simulink model "SimplifiedShiftController5"  (Simulink 8.2)
settings: Solver=ode45  StartTime=0.0  StopTime=10.0  RelTol=1e-3
settings Model: Creator=root  LastModifiedBy=tiwari
settings DataIOCC: SignalLoggingSaveFormat=Dataset
settings OptimizationCC: ExpressionDepthLimit=128
settings DebuggingCC: FcnCallInpInsideContextMsg=EnableAllAsError
settings GRTTargetCC: CombineOutputUpdateFcns=on  GRTInterface=off

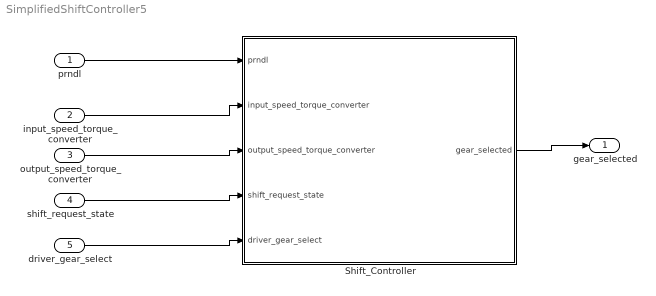
== system SimplifiedShiftController5 ==
  prndl : Inport
  input_speed_torque_converter : Inport  Port=2
  output_speed_torque_converter : Inport  Port=3
  shift_request_state : Inport  Port=4
  driver_gear_select : Inport  Port=5
  Shift_Controller : Subsystem
  gear_selected : Outport
  wires:
  prndl/1 -> Shift_Controller/1(prndl)
  shift_request_state/1 -> Shift_Controller/4(shift_request_state)
  driver_gear_select/1 -> Shift_Controller/5(driver_gear_select)
  output_speed_torque_converter/1 -> Shift_Controller/3(output_speed_torque_converter)
  input_speed_torque_converter/1 -> Shift_Controller/2(input_speed_torque_converter)
  Shift_Controller/1(gear_selected) -> gear_selected/1

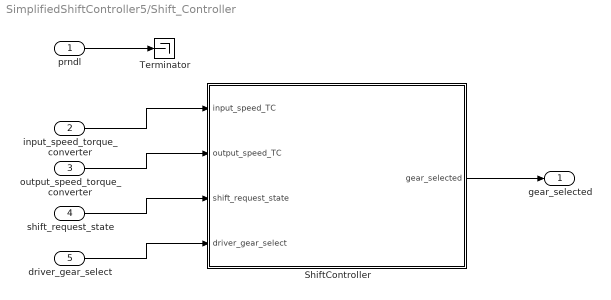
== system SimplifiedShiftController5/Shift_Controller ==
  prndl : Inport
  input_speed_torque_converter : Inport  Port=2
  output_speed_torque_converter : Inport  Port=3
  shift_request_state : Inport  Port=4
  driver_gear_select : Inport  Port=5
  ShiftController : Stateflow chart  TreatAsAtomicUnit=on
  Terminator : Terminator
  gear_selected : Outport
  wires:
  ShiftController/1(gear_selected) -> gear_selected/1
  prndl/1 -> Terminator/1
  input_speed_torque_converter/1 -> ShiftController/1(input_speed_TC)
  output_speed_torque_converter/1 -> ShiftController/2(output_speed_TC)
  shift_request_state/1 -> ShiftController/3(shift_request_state)
  driver_gear_select/1 -> ShiftController/4(driver_gear_select)

== stateflow chart Shift_Controller/ShiftController ==
  settings: description=|
      | <?xml version="1.0" encoding="utf-8"?>
      | <ltlProperties>
      |    <ltlProperty expr="&lt;&gt;((driver_gear_select==6 || driver_gear_select==7)) -&gt; (!((gear_selected /= 0)) U((driver_gear_select==6 || driver_gear_select==7)))" name="AbsenceProperty" type="Absence"/>
      |    <ltlProperty expr="[]((driver_gear_select==6) -&gt; &lt;&gt;(gear_selected &gt;= 1))" name="ResponseProperty" type="Response"/>
      |    <ltlProperty expr="[](((shift_request_state==3 &amp;&amp; driver_gear_select==7)) -&gt; &lt;&gt;(gear_selected == 4))" name="ResponseProperty2" type="Response"/>
      |    <ltlProperty expr="[]((G(shift_request_state==3 &amp;&amp; driver_gear_select==7)) -&gt; &lt;&gt;((gear_selected == 4)))" name="ResponseProperty3" type="Response"/>
      |    <ltlProperty expr="[]((G(driver_gear_select == 1)) -&gt; &lt;&gt;((gear_selected &lt;= 1)))" name="ResponseProperty4" type="Response"/>
      |    <ltlProperty expr="[]((G(driver_gear_select==1)) -&gt; &lt;&gt;((gear_selected &lt;= 2)))" name="ResponseProperty5" type="Response"/>
      | </ltlProperties>
  state gear1
    en:gear_selected=1;
  state lockoutU2
    en: current_time = 0;
    du: current_time += SamplePeriod;
  state gear2
    en: gear_selected = 2;
  state lockoutD1
    en: current_time = 0;
    du: current_time += SamplePeriod;
  state lockoutD2
    en: current_time = 0;
    du: current_time += SamplePeriod;
  state lockoutD3
    en: current_time = 0;
    du: current_time += SamplePeriod;
  state lockoutU3
    en: current_time = 0;
    du: current_time += SamplePeriod;
  state lockoutU4
    en: current_time = 0;
    du:current_time += SamplePeriod;
  state gear3
    en: gear_selected = 3;
  state gear4
    en: gear_selected = 4;
  state gear0
    en:gear_selected=0;
  (default) -> gear0
  gear0 -> gear1 : [(driver_gear_select==6)||(driver_gear_select==7)]
  lockoutD1 -> gear1 : [current_time >= lockout_time]
  gear1 -> lockoutU2 : [(shift_request_state == 3) && (driver_gear_select != 6) && (driver_gear_select != 1)]
  lockoutU2 -> gear2 : [current_time >= lockout_time]
  gear3 -> lockoutD1 [order 3] : [(driver_gear_select == 6) || (driver_gear_select == 1)]
  gear4 -> lockoutD1 [order 2] : [(driver_gear_select == 6) || (driver_gear_select == 1)]
  gear2 -> lockoutD1 [order 2] : [((shift_request_state == 1) && (driver_gear_select != 6) && (driver_gear_select != 1) && (input_speed_TC > output_speed_TC)) || (driver_gear_select==6) || (driver_gear_select==1)]
  lockoutD2 -> gear2 : [current_time >= lockout_time]
  gear2 -> lockoutU3 [order 1] : [(shift_request_state == 3) && (driver_gear_select != 6) && (driver_gear_select != 1)]
  gear3 -> lockoutD2 [order 2] : [(shift_request_state == 1) && (driver_gear_select != 6) && (driver_gear_select != 1) && (input_speed_TC > output_speed_TC)]
  lockoutU3 -> gear3 : [current_time >= lockout_time]
  lockoutD3 -> gear3 : [current_time >= lockout_time]
  gear3 -> lockoutU4 [order 1] : [(shift_request_state == 3) && (driver_gear_select != 6) && (driver_gear_select != 1)]
  gear4 -> lockoutD3 [order 1] : [(shift_request_state == 1) && (driver_gear_select != 6) && (driver_gear_select != 1) && (input_speed_TC > output_speed_TC)]
  lockoutU4 -> gear4 : [current_time >= lockout_time]
  data: input_speed_TC input double; output_speed_TC input double; shift_request_state input int32; driver_gear_select input int32; gear_selected output int32; lockout_time local double; current_time local double; SamplePeriod local double =0.01; dummy local double
